simulink model "Corner_Light_Sfunction"  (R2020a)
settings: Solver=FixedStepDiscrete  StartTime=0.0  StopTime=10.0  FixedStep=1  RelTol=1e-3
settings Model: Creator=hp  LastModifiedBy=hp
settings DataIOCC: SaveOutput=off  SaveTime=off
settings OptimizationCC: DefaultParameterBehavior=Inlined
settings ConfigComp: CovMetricSettings=dcmwe

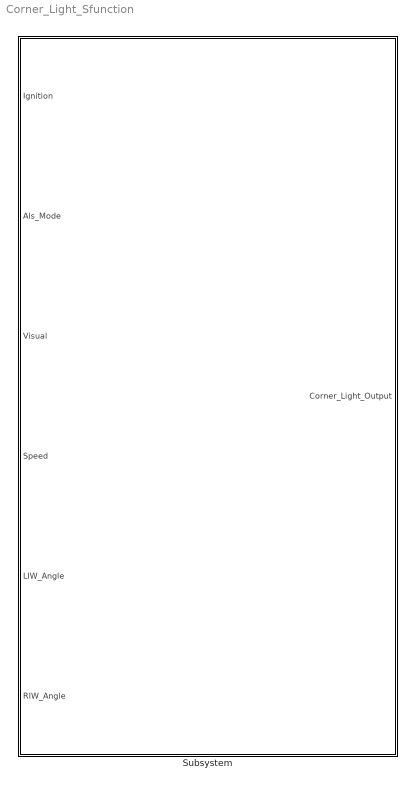
== system Corner_Light_Sfunction ==
  Subsystem : Subsystem
      mask help: Simulink:masks:GenSFuncDesc_MD
      mask Help: eval('feval(''rtwprivate'',''rtwhelpview'',''rtw_sfcn_block'')');

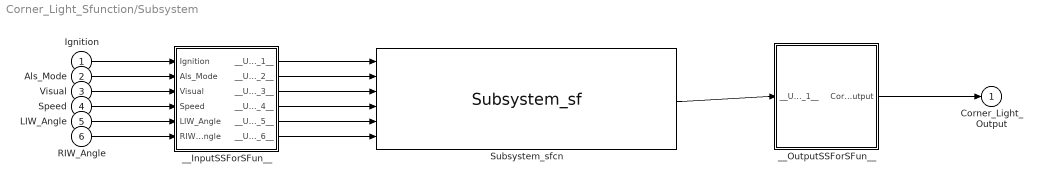
== system Corner_Light_Sfunction/Subsystem ==
  Ignition : Inport
  Als_Mode : Inport  Port=2
  Visual : Inport  Port=3
  Speed : Inport  Port=4
  LIW_Angle : Inport  Port=5
  RIW_Angle : Inport  Port=6
  Subsystem_sfcn : S-Function  FunctionName=Subsystem_sf  SFunctionModules=""  SFunctionDeploymentMode=off  EnableBusSupport=off  mask{rtw_sf_name=Subsystem_sf, showVar=off}
      mask prompts: rtw_sf_name "Simulink:masks:GenSFuncName_MP"; showVar "Simulink:masks:GenSFuncShowModuleList_MP"
      mask help: Simulink:masks:GenSFuncDesc_MD
      mask init:
      | displist = '';
      | if ~strcmp(get_param(gcb, 'FunctionName'), rtw_sf_name);
      |   set_param(gcb, 'FunctionName', rtw_sf_name);
      | end
      | % Check if we are generating code
      | rtw_mode = false;
      | if strcmpi(get_param(bdroot(gcb),'SimulationStatus'),'Initializing')
      | 	rtw_mode = strcmpi(get_param(bdroot(gcb),'BuildingRTWCode'),'on') && ...
      | 		~strcmpi(get_param(bdroot(gcb),'TargetStyle'),'SimulationTarget');
      | end
      | if showVar || rtw_mode
      | 	if exist('rtwsfunc') == 2 | exist('rtwsfunc') == 6
      | 		tmplist = rtwsfunc(rtw_sf_name,gcb);
      | 		tmplist = DAStudio.message('Simulink:masks:GenSFuncListOfModules_IC', tmplist);
      | 	elseif showVar
      | 		tmplist1 = DAStudio.message('Simulink:masks:GenSFuncListOfModules_IC', '');
      |         tmplist2 = DAStudio.message('Simulink:masks:GenSFuncNotLicensed_IC');
      |         tmplist = [tmplist1 tmplist2];
      |  	end
      | end
      | if showVar
      |   displist = tmplist;
      | end
      settings: CopyFcn=|
      | if ~strcmp(get_param(gcb,'Linkstatus'),'none') && ...
      | ~strcmp(get_param(gcb,'Linkstatus'),'implicit')
      |   set_param(gcb,'LinkStatus','none');
      | end
      mask Help: eval('feval(''rtwprivate'',''rtwhelpview'',''rtw_sfcn_block'')');
      mask Display:
      | port_label('input',1,'Ignition');
      | port_label('input',2,'Als_Mode');
      | port_label('input',3,'Visual');
      | port_label('input',4,'Speed');
      | port_label('input',5,'LIW_Angle');
      | port_label('input',6,'RIW_Angle');
      | port_label('output',1,'Corner_Light_Output');
  __InputSSForSFun__ : Subsystem
  __OutputSSForSFun__ : Subsystem
  Corner_Light_Output : Outport
  wires:
  Ignition/1 -> __InputSSForSFun__/1(Ignition)
  Als_Mode/1 -> __InputSSForSFun__/2(Als_Mode)
  Visual/1 -> __InputSSForSFun__/3(Visual)
  Speed/1 -> __InputSSForSFun__/4(Speed)
  LIW_Angle/1 -> __InputSSForSFun__/5(LIW_Angle)
  RIW_Angle/1 -> __InputSSForSFun__/6(RIW_Angle)
  __InputSSForSFun__/1(__UniqueOutportName__1__) -> Subsystem_sfcn/1
  __InputSSForSFun__/2(__UniqueOutportName__2__) -> Subsystem_sfcn/2
  __InputSSForSFun__/3(__UniqueOutportName__3__) -> Subsystem_sfcn/3
  __InputSSForSFun__/4(__UniqueOutportName__4__) -> Subsystem_sfcn/4
  __InputSSForSFun__/5(__UniqueOutportName__5__) -> Subsystem_sfcn/5
  __InputSSForSFun__/6(__UniqueOutportName__6__) -> Subsystem_sfcn/6
  Subsystem_sfcn/1 -> __OutputSSForSFun__/1(__UniqueInportName__1__)
  __OutputSSForSFun__/1(Corner_Light_Output) -> Corner_Light_Output/1

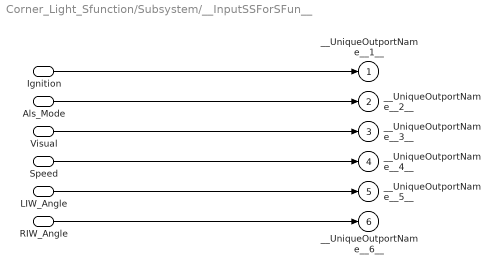
== system Corner_Light_Sfunction/Subsystem/__InputSSForSFun__ ==
  Ignition : Inport
  Als_Mode : Inport  Port=2
  Visual : Inport  Port=3
  Speed : Inport  Port=4
  LIW_Angle : Inport  Port=5
  RIW_Angle : Inport  Port=6
  __UniqueOutportName__1__ : Outport
  __UniqueOutportName__2__ : Outport  Port=2
  __UniqueOutportName__3__ : Outport  Port=3
  __UniqueOutportName__4__ : Outport  Port=4
  __UniqueOutportName__5__ : Outport  Port=5
  __UniqueOutportName__6__ : Outport  Port=6
  wires:
  Ignition/1 -> __UniqueOutportName__1__/1
  Als_Mode/1 -> __UniqueOutportName__2__/1
  Visual/1 -> __UniqueOutportName__3__/1
  Speed/1 -> __UniqueOutportName__4__/1
  LIW_Angle/1 -> __UniqueOutportName__5__/1
  RIW_Angle/1 -> __UniqueOutportName__6__/1

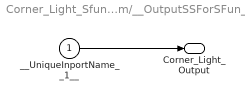
== system Corner_Light_Sfunction/Subsystem/__OutputSSForSFun__ ==
  __UniqueInportName__1__ : Inport
  Corner_Light_Output : Outport
  wires:
  __UniqueInportName__1__/1 -> Corner_Light_Output/1
